simulink model "feedforwad"  (R2023a)
settings: Solver=VariableStepAuto  StartTime=0.0  StopTime=10.0  RelTol=1e-3
values from neighbouring files (symbols this model uses):
  feed_forward_gain = 1 / G_0    (= 1.26582278481)    [project.m]
  K_lag = 1    [project.m]
  K_lead = 5    [project.m]
  K_lead_0 = K_lead / alpha    (= 12.5)    [project.m]
  K_lead_initial = 1    [project.m]
settings Model: Creator=ye  LastModifiedBy=ye

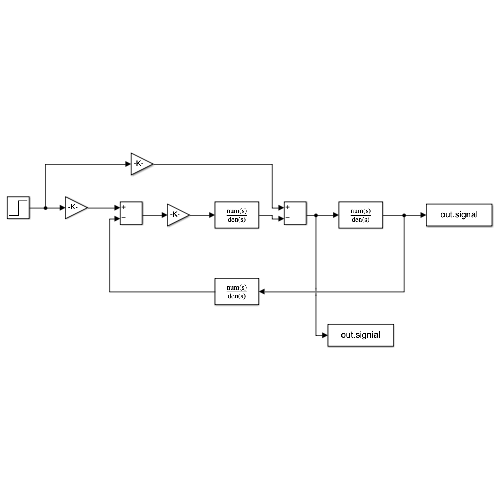
[thumbnail: Simulink's stored preview of the top-level diagram]
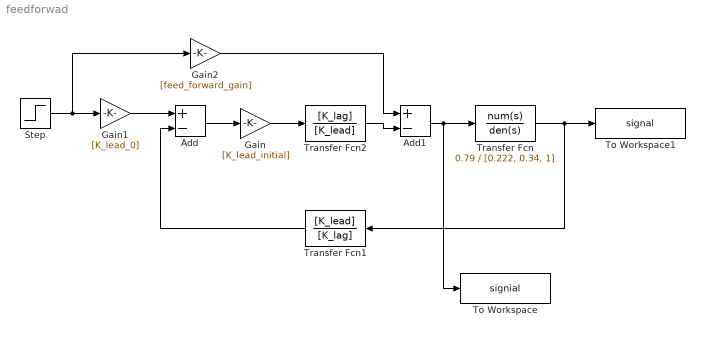
== system feedforwad ==
  Add : Sum  Inputs=+-
  Add1 : Sum  Inputs=+-
  Gain : Gain  Gain=[K_lead_initial]
  Gain1 : Gain  Gain=[K_lead_0]
  Gain2 : Gain  Gain=[feed_forward_gain]
  Step : Step  SampleTime=0
  To Workspace : ToWorkspace  VariableName=signial  SaveFormat=Timeseries  SampleTime=-1
  To Workspace1 : ToWorkspace  VariableName=signal  SaveFormat=Timeseries  SampleTime=-1
  Transfer Fcn : TransferFcn  Numerator=0.79  Denominator=[0.222, 0.34, 1]
  Transfer Fcn1 : TransferFcn  Numerator=[K_lead]  Denominator=[K_lag]
  Transfer Fcn2 : TransferFcn  Numerator=[K_lag]  Denominator=[K_lead]
  wires:
  Gain1/1 -> Add/1
  Transfer Fcn/1 -> Transfer Fcn1/1, To Workspace1/1
  Gain/1 -> Transfer Fcn2/1
  Add/1 -> Gain/1
  Transfer Fcn1/1 -> Add/2
  Step/1 -> Gain2/1, Gain1/1
  Gain2/1 -> Add1/1
  Transfer Fcn2/1 -> Add1/2
  Add1/1 -> To Workspace/1, Transfer Fcn/1
